simulink model "Sim_AllDifferentiator"  (R2021a)
settings: Solver=VariableStepAuto  StartTime=ti  StopTime=tf  RelTol=1e-3
values from neighbouring files (symbols this model uses):
  a = 2    [InitParams.m]
  alpha = paramsnHomD.alpha    [nHomD.m]    (also in nHomDR.m = paramsnHomDR.alpha)
  gain = paramsnHGD.gain    [nHGD.m]    (also in nHGDR.m = paramsnHGDR.gain; nHOSMD.m = paramsnHOSMD.gain; nHomD.m = paramsnHomD.gain; nHomDR.m = paramsnHomDR.gain)
  k = 1    [InitParams.m]
  n = 1    [InitParams.m]    (also in nFxTHomDR.m = paramsnFxTHomDR.n; nHGD.m = paramsnHGD.n; nHGDR.m = paramsnHGDR.n; nHOSMD.m = paramsnHOSMD.n)
  omega = 2    [InitParams.m]
  theta = paramsnHGD.theta    [nHGD.m]    (also in nHGDR.m = paramsnHGDR.theta; nHOSMD.m = paramsnHOSMD.theta; nHomD.m = paramsnHomD.theta; nHomDR.m = paramsnHomDR.theta)
undefined symbols (not defined in the file or in its folder): Noise, tau
libraries: simulink x1
settings Model: Creator=perruquetti  LastModifiedBy=perruquetti
settings SolverCC: AlgebraicLoopSolver=TrustRegion
settings DataIOCC: ReturnWorkspaceOutputs=off
settings DebuggingCC: SFMachineParentedDataDiag=warning  ArithmeticOperatorsInVariantConditions=warning
settings SFSimCC: SimUseLocalCustomCode=off  CustomCodeUndefinedFunction=UseInterfaceOnly
settings RTWCC: RTWUseLocalCustomCode=off

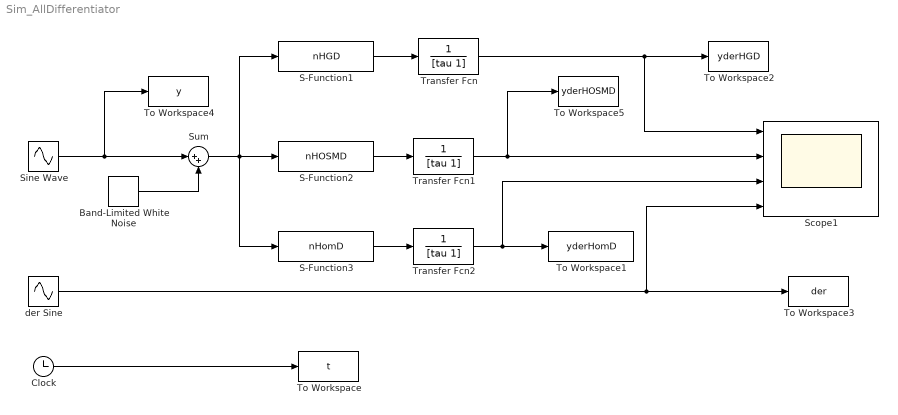
== system Sim_AllDifferentiator ==
  Band-Limited White Noise : simulink/Sources/Band-Limited White Noise  Cov=Noise.power  Ts=Noise.sampling  seed=Noise.seed
  Clock : Clock
  S-Function1 : S-Function  FunctionName=nHGD  Parameters=n,gain,theta  SFunctionDeploymentMode=off  EnableBusSupport=off
  S-Function2 : S-Function  FunctionName=nHOSMD  Parameters=n,gain,theta  SFunctionDeploymentMode=off  EnableBusSupport=off
  S-Function3 : S-Function  FunctionName=nHomD  Parameters=n,gain,theta,alpha  SFunctionDeploymentMode=off  EnableBusSupport=off
  Scope1 : Scope  NumInputPorts=4
  Sine Wave : Sin  Amplitude=a  Frequency=omega  SampleTime=0
  Sum : Sum  Inputs=|++
  To Workspace : ToWorkspace  VariableName=t  SampleTime=-1
  To Workspace1 : ToWorkspace  VariableName=yderHomD  SampleTime=-1
  To Workspace2 : ToWorkspace  VariableName=yderHGD  SampleTime=-1
  To Workspace3 : ToWorkspace  VariableName=der  SampleTime=-1
  To Workspace4 : ToWorkspace  VariableName=y  SampleTime=-1
  To Workspace5 : ToWorkspace  VariableName=yderHOSMD  SampleTime=-1
  Transfer Fcn : TransferFcn  Denominator=[tau 1]
  Transfer Fcn1 : TransferFcn  Denominator=[tau 1]
  Transfer Fcn2 : TransferFcn  Denominator=[tau 1]
  der Sine : Sin  Amplitude=a*omega^k  Frequency=omega  Phase=k*pi/2  SampleTime=0
  wires:
  Clock/1 -> To Workspace/1
  Sine Wave/1 -> To Workspace4/1, Sum/1
  S-Function1/1 -> Transfer Fcn/1
  Band-Limited White Noise/1 -> Sum/2
  Sum/1 -> S-Function1/1, S-Function3/1, S-Function2/1
  S-Function2/1 -> Transfer Fcn1/1
  S-Function3/1 -> Transfer Fcn2/1
  der Sine/1 -> Scope1/4, To Workspace3/1
  Transfer Fcn/1 -> To Workspace2/1, Scope1/1
  Transfer Fcn1/1 -> To Workspace5/1, Scope1/2
  Transfer Fcn2/1 -> Scope1/3, To Workspace1/1
